simulink model "CH22_6C"  (Simulink 10.1)
settings: Solver=ode45  StartTime=0.0  StopTime=inf  RelTol=1e-3  EnableMultiTasking=on
undefined symbols (not defined in the file or in its folder): gcbh, rcfiltgaincompat
libraries: commrandsrc2 x2, commfilt2 x2, commutil2 x2
settings Model: Creator=my2  LastModifiedBy=IT
settings DataIOCC: LimitDataPoints=on  SignalLoggingSaveFormat=ModelDataLogs
settings DebuggingCC: SolverPrmCheckMsg=warning  MultiTaskDSMMsg=warning  MultiTaskCondExecSysMsg=none  FcnCallInpInsideContextMsg=warning

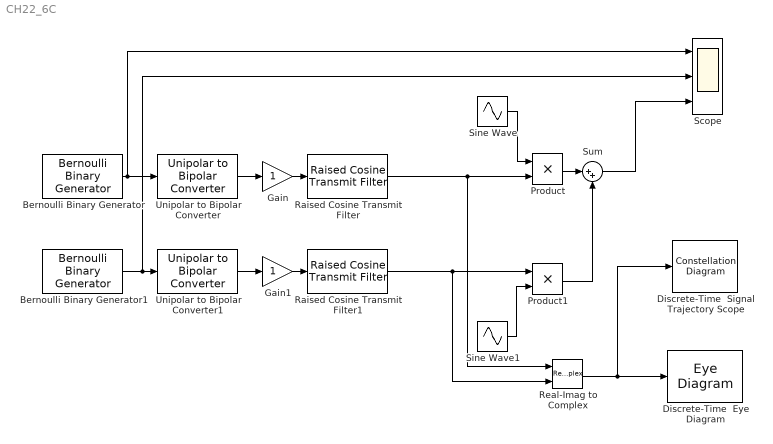
== system CH22_6C ==
  Bernoulli Binary Generator : commrandsrc2/Bernoulli Binary Generator  P=0.5  seed=71  Ts=1  frameBased=off  sampPerFrame=1  orient=off  outDataType=boolean
      settings: SourceProductBaseCode=CM
  Bernoulli Binary Generator1 : commrandsrc2/Bernoulli Binary Generator  P=0.5  seed=61  Ts=1  frameBased=off  sampPerFrame=1  orient=off  outDataType=boolean
      settings: SourceProductBaseCode=CM
  Discrete-Time  Eye Diagram : EyeDiagram  Tag=EyeDiagram
  Discrete-Time  Signal Trajectory Scope : ConstellationDiagram  Tag=ScatterPlot
  Gain : Gain
  Gain1 : Gain
  Product : Product
  Product1 : Product
  Raised Cosine Transmit Filter : commfilt2/Raised Cosine Transmit Filter  filtType=Square root  R=0.75  filtSpan=2*(5)  N=256  filterGain=rcfiltgaincompat(gcbh)  RateOptions=Allow multirate processing  framing=Mute  checkCoeff=off  variableName=rcTxFilt  checkGain=Normalized  sampMode=Mute  saveAsFlag=0  currentFiltSpan=2*(5)  D=5  launchFVT=on  roundingMode=Floor  overflowMode=off  coeffDataTypeStr=Inherit: Same word length as input  coeffMin=[]  coeffMax=[]  coeffLastDataTypeStr=Inherit: Same word length as input  outputDataTypeStr=Inherit: Same as accumulator  outputMin=[]  outputMax=[]  outputLastDataTypeStr=Inherit: Same as accumulator
  Raised Cosine Transmit Filter1 : commfilt2/Raised Cosine Transmit Filter  filtType=Square root  R=0.75  filtSpan=2*(5)  N=256  filterGain=rcfiltgaincompat(gcbh)  RateOptions=Allow multirate processing  framing=Mute  checkCoeff=off  variableName=rcTxFilt1  checkGain=Normalized  sampMode=Mute  saveAsFlag=0  currentFiltSpan=2*(5)  D=5  launchFVT=on  roundingMode=Floor  overflowMode=off  coeffDataTypeStr=Inherit: Same word length as input  coeffMin=[]  coeffMax=[]  coeffLastDataTypeStr=Inherit: Same word length as input  outputDataTypeStr=Inherit: Same as accumulator  outputMin=[]  outputMax=[]  outputLastDataTypeStr=Inherit: Same as accumulator
  Real-Imag to Complex : RealImagToComplex
  Scope : Scope  NumInputPorts=3
  Sine Wave : Sin  SampleTime=1/256
  Sine Wave1 : Sin  SampleTime=1/256
  Sum : Sum  Inputs=|++
  Unipolar to Bipolar Converter : commutil2/Unipolar to Bipolar Converter  M=2  polarity=Positive  dataType=Inherit via internal rule
  Unipolar to Bipolar Converter1 : commutil2/Unipolar to Bipolar Converter  M=2  polarity=Positive  dataType=Inherit via internal rule
  wires:
  Bernoulli Binary Generator/1 -> Scope/1, Unipolar to Bipolar Converter/1
  Unipolar to Bipolar Converter/1 -> Gain/1
  Bernoulli Binary Generator1/1 -> Scope/2, Unipolar to Bipolar Converter1/1
  Unipolar to Bipolar Converter1/1 -> Gain1/1
  Sine Wave/1 -> Product/1
  Gain/1 -> Raised Cosine Transmit Filter/1
  Gain1/1 -> Raised Cosine Transmit Filter1/1
  Sine Wave1/1 -> Product1/2
  Product/1 -> Sum/1
  Product1/1 -> Sum/2
  Sum/1 -> Scope/3
  Raised Cosine Transmit Filter/1 -> Product/2, Real-Imag to Complex/1
  Real-Imag to Complex/1 -> Discrete-Time  Signal Trajectory Scope/1, Discrete-Time  Eye Diagram/1
  Raised Cosine Transmit Filter1/1 -> Product1/1, Real-Imag to Complex/2
